simulink model "sm_aileron_actuator_mech_01_ail"  (R2023b)
settings: Solver=VariableStepAuto  StartTime=0.0  StopTime=10.0  RelTol=1e-3  EnableMultiTasking=on
PreLoadFcn:
  | aileronAssembly_DataFile
undefined symbols (not defined in the file): AAC_Param, actbase_x, actbase_y, smiData, X, Y, Z
libraries: sm_lib x303, nesl_utility x1
(part 1 of 6)
Description:
  | Copyright 2018-2022 The MathWorks, Inc.
settings Model: Creator=smiller  LastModifiedBy=mkhaleghi
settings SolverCC: AlgebraicLoopSolver=TrustRegion
settings DataIOCC: LimitDataPoints=on
settings OptimizationCC: ReuseModelBlockBuffer=off  LifeSpan=inf
settings DebuggingCC: UnconnectedInputMsg=warning  UnconnectedOutputMsg=warning  UnconnectedLineMsg=warning  AllowSymbolicDim=off  PregeneratedLibrarySubsystemCodeDiagnostic=none  SFUnexpectedBacktrackingDiag=warning  SFNoUnconditionalDefaultTransitionDiag=warning  SFExecutionAtInitializationDiag=none  ArithmeticOperatorsInVariantConditions=warning
settings ModelReferenceCC: EnableRefExpFcnMdlSchedulingChecks=on
settings SFSimCC: SimUseLocalCustomCode=off  CustomCodeUndefinedFunction=UseInterfaceOnly
settings RTWCC: RTWUseLocalCustomCode=off  DLArmComputeVersion=19.05
settings CodeAppCC: StateflowObjectComments=on
settings GRTTargetCC: TargetLangStandard=C89/C90 (ANSI)
settings ConfigComp: CovMetricSettings=dw  CovSaveCumulativeToWorkspaceVar=on  CovSaveSingleToWorkspaceVar=on  CovExternalEMLEnable=off  CovSFcnEnable=off
settings SimscapeCC: SimscapeNominalValues="[{\"value\":\"10\",\"unit\":\"V\"},{\"value\":\"1\",\"unit\":\"A\"},{\"value\":\"10\",\"unit\":\"N*m\"},{\"value\":\"10\",\"unit\":\"bar\"},{\"value\":\"100\",\"unit\":\"kJ/kg\"},{\"value\":\"1\",\"unit\":\"kW\"},{\"value\":\"300\",\"unit\":\"K\"},{\"value\":\"100\",\"unit\":\"cm^3/s\"},{\"value\":\"1\",\"unit\":\"kN\"},{\"value\":\"1\",\"unit\":\"g/cm^3\"},{\"value\":\"1\",\"unit\":\"l\"},{\"value\":\"1\",\"unit\":\"cm^2\"},{\"value\":\"60\",\"unit\":\"Hz\"}]"  SimscapeLogType=all  SimscapeLogDataHistory=10000
settings ConfigurationSet: Description=SimMechanics 2G
settings ExplorerConfigSet: InternalSimMechanicsExplorerSettings="<ExplorerConfiguration><canonicalview>default</canonicalview><AnimationSetting><BasePlaybackSpeed>1.0</BasePlaybackSpeed><PlaybackSpeedFactor>1.0</PlaybackSpeedFactor></AnimationSetting><TilePanel><TileInfo><Tiles Columns=\"1\" Count=\"1\" Rows=\"1\"><Column Weight=\"1\"/><Row Weight=\"1\"/><Tile Height=\"1\" Width=\"1\" X=\"0\" Y=\"0\"/></Tiles></TileInfo><SceneInfo><SceneViewer><BGColor><R>1</R><G>1</G><B>1</B></BGColor><Camera><DoPerspective>off</DoPerspective><Position><X>0.188789670070064197</X><Y>0.0456123314797882706</Y><Z>3.03630010044172227</Z></Position><Center><X>0.188789670070064197</X><Y>0.0456123314797882706</Y><Z>-0.0389997633735852389</Z></Center><Up><X>0</X><Y>1</Y><Z>-0</Z></Up><ViewLimDist>1</ViewLimDist><YLim>0.256282721906246236</YLim><XLim>0.407121367156505543</XLim></Camera></SceneViewer></SceneInfo></TilePanel><MechEditorPanel><Cameras/><GfxPanelCameraMap/><VideoCreator><PlaybackSpeedRatio>1.0</PlaybackSpeedRatio><FrameRate>30</FrameRate><VideoFormat>Motion JPEG AVI</VideoFormat><FrameSize>auto</FrameSize></VideoCreator></MechEditorPanel></ExplorerConfiguration>"

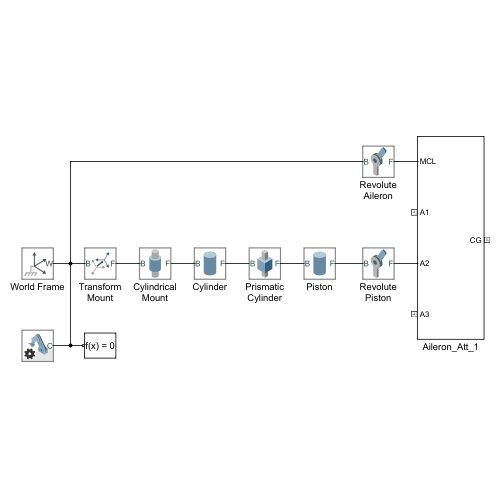
[thumbnail: Simulink's stored preview of the top-level diagram]
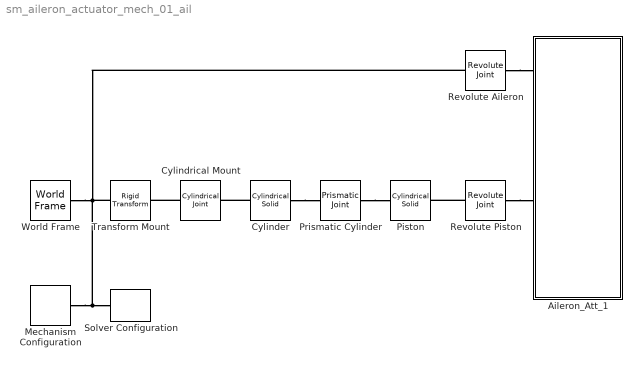
== system sm_aileron_actuator_mech_01_ail ==
  Aileron_Att_1 : Subsystem  RequirementInfo={} %GIDa_f86a7f46_afc1_4b35_ab70_400c1aa97c7d
  Cylinder : sm_lib/Body Elements/Cylindrical Solid  GraphicAmbientColor=[0.15 0.15 0.15 1.0]  BasedOnType=Density  CenterOfMass=[0 0 0]  CenterOfMassUnits=m  GraphicDiffuseColor=[1.0 0.8 0.4]  CylinderLength=cyl_length  CylinderLengthUnits=m  CylinderRadius=cyl_radius  CylinderRadiusUnits=m  Density=1000  DensityUnits=kg/m^3  DoExposeReferenceFrame=off  GraphicEmissiveColor=[0.0 0.0 0.0 1.0]  ExportEntireGeometry=off  SerializedFrames=<Frames><Frame><Id>Frame1</Id><Value><Name>F</Name><Origin><Source>GeometricFeature</Source><FeatureName>top surface</FeatureName></Origin><PrimaryAxis><DefinedDirection>+Z</DefinedDirection><Source>GeometricFeature</Source><SourceDirection>+Z</SourceDirection><FeatureName>top surface</FeatureName></PrimaryAxis><SecondaryAxis><DefinedDirection>+X</DefinedDirection><Source>ReferenceFrame</Source><SourceDirection>+X</SourceDirection><FeatureName></FeatureName></SecondaryAxis></Value></Frame><Frame><Id>Frame2</Id><Value><Name>B</Name><Origin><Source>GeometricFeature</Source><FeatureName>bottom surface</FeatureName></Origin><PrimaryAxis><DefinedDirection>+Z</DefinedDirection><Source>ReferenceFrame</Source><SourceDirection>-X</SourceDirection><FeatureName></FeatureName></PrimaryAxis><SecondaryAxis><DefinedDirection>+X</DefinedDirection><Source>ReferenceFrame</Source><SourceDirection>+Z</SourceDirection><FeatureName></FeatureName></SecondaryAxis></Value></Frame></Frames>  MarkerShape=Sphere  MarkerSize=10  GraphicType=FromGeometry  InertiaType=CalculateFromGeometry  Mass=1  MassUnits=kg  MomentsOfInertia=[1 1 1]  MomentsOfInertiaUnits=kg*m^2  GraphicOpacity=1.0  ProductsOfInertia=[0 0 0]  ProductsOfInertiaUnits=kg*m^2  GraphicShininess=75  GraphicSpecularColor=[0.5 0.5 0.5 1.0]  GraphicVisPropType=SimpleVisualProperties
  Cylindrical Mount : sm_lib/Joints/Cylindrical Joint  JointMode=Normal  SenseConstraintForce=off  SenseConstraintForceX=off  SenseConstraintForceY=off  SenseConstraintForceZ=off  SenseConstraintTorque=off  SenseConstraintTorqueX=off  SenseConstraintTorqueY=off  SenseConstraintTorqueZ=off  SenseTotalForce=off  SenseTotalForceX=off  SenseTotalForceY=off  SenseTotalForceZ=off  SenseTotalTorque=off  SenseTotalTorqueX=off  SenseTotalTorqueY=off  SenseTotalTorqueZ=off  CompositeWrenchDir=FollowerOnBase  CompositeWrenchFrame=BaseFrame  PzEquilibriumPosition=0  PzEquilibriumPositionUnits=m  PzSpringStiffness=0  PzSpringStiffnessUnits=N/m  PzDampingCoefficient=0  PzDampingCoefficientUnits=N/(m/s)  PzTorqueActuationMode=NoTorque  PzMotionActuationMode=ComputedMotion  PzSensePosition=off  PzSenseVelocity=off  PzSenseAcceleration=off  PzSenseTorqueForce=off  PzSenseLowerLimitTorqueForce=off  PzSenseUpperLimitTorqueForce=off  PzLowerLimitSpecify=off  PzLowerLimitBound=-1  PzLowerLimitBoundUnits=m  PzLowerLimitStiffness=1e6  PzLowerLimitStiffnessUnits=N/m  PzLowerLimitDamping=1e3  PzLowerLimitDampingUnits=N/(m/s)  PzLowerLimitTransitionRegionWidth=1e-4  PzLowerLimitTransitionRegionWidthUnits=m  PzUpperLimitSpecify=off  PzUpperLimitBound=1  PzUpperLimitBoundUnits=m  PzUpperLimitStiffness=1e6  PzUpperLimitStiffnessUnits=N/m  PzUpperLimitDamping=1e3  PzUpperLimitDampingUnits=N/(m/s)  PzUpperLimitTransitionRegionWidth=1e-4  PzUpperLimitTransitionRegionWidthUnits=m  PzPositionTargetSpecify=off  PzPositionTargetPriority=High  PzPositionTargetValue=0  PzPositionTargetValueUnits=m  PzVelocityTargetSpecify=off  PzVelocityTargetPriority=High  PzVelocityTargetValue=0  PzVelocityTargetValueUnits=m/s  RzEquilibriumPosition=0  RzEquilibriumPositionUnits=deg  RzSpringStiffness=0  RzSpringStiffnessUnits=N*m/deg  RzDampingCoefficient=0  RzDampingCoefficientUnits=N*m/(deg/s)  RzTorqueActuationMode=NoTorque  RzMotionActuationMode=ComputedMotion  RzSensePosition=off  RzSenseVelocity=off  RzSenseAcceleration=off  RzSenseTorqueForce=off  RzSenseLowerLimitTorqueForce=off  RzSenseUpperLimitTorqueForce=off  RzLowerLimitSpecify=off  RzLowerLimitBound=-90  RzLowerLimitBoundUnits=deg  RzLowerLimitStiffness=1e4  RzLowerLimitStiffnessUnits=N*m/deg  RzLowerLimitDamping=10  RzLowerLimitDampingUnits=N*m/(deg/s)  RzLowerLimitTransitionRegionWidth=0.1  RzLowerLimitTransitionRegionWidthUnits=deg  RzUpperLimitSpecify=off  RzUpperLimitBound=90  RzUpperLimitBoundUnits=deg  RzUpperLimitStiffness=1e4  RzUpperLimitStiffnessUnits=N*m/deg  RzUpperLimitDamping=10  RzUpperLimitDampingUnits=N*m/(deg/s)  RzUpperLimitTransitionRegionWidth=0.1  RzUpperLimitTransitionRegionWidthUnits=deg  RzPositionTargetSpecify=off  RzPositionTargetPriority=High  RzPositionTargetValue=0  RzPositionTargetValueUnits=deg  RzVelocityTargetSpecify=off  RzVelocityTargetPriority=High  RzVelocityTargetValue=0  RzVelocityTargetValueUnits=deg/s
  Mechanism Configuration : sm_lib/Utilities/Mechanism Configuration  UniformGravity=Constant  GravityVector=[0 -9.80665 0]  GravityVectorUnits=m/s^2  LinearizationDelta=0.001  JointModeTransitionNonlinearIterations=2
  Piston : sm_lib/Body Elements/Cylindrical Solid  GraphicAmbientColor=[0.15 0.15 0.15 1.0]  BasedOnType=Density  CenterOfMass=[0 0 0]  CenterOfMassUnits=m  GraphicDiffuseColor=[0.5 0.5 0.5]  CylinderLength=piston_length  CylinderLengthUnits=m  CylinderRadius=piston_radius  CylinderRadiusUnits=m  Density=1000  DensityUnits=kg/m^3  DoExposeReferenceFrame=off  GraphicEmissiveColor=[0.0 0.0 0.0 1.0]  ExportEntireGeometry=off  SerializedFrames=<Frames><Frame><Id>Frame1</Id><Value><Name>F</Name><Origin><Source>GeometricFeature</Source><FeatureName>top surface</FeatureName></Origin><PrimaryAxis><DefinedDirection>+Z</DefinedDirection><Source>ReferenceFrame</Source><SourceDirection>-X</SourceDirection><FeatureName></FeatureName></PrimaryAxis><SecondaryAxis><DefinedDirection>+X</DefinedDirection><Source>ReferenceFrame</Source><SourceDirection>+Z</SourceDirection><FeatureName></FeatureName></SecondaryAxis></Value></Frame><Frame><Id>Frame2</Id><Value><Name>B</Name><Origin><Source>GeometricFeature</Source><FeatureName>bottom surface</FeatureName></Origin><PrimaryAxis><DefinedDirection>+Z</DefinedDirection><Source>ReferenceFrame</Source><SourceDirection>+Z</SourceDirection><FeatureName></FeatureName></PrimaryAxis><SecondaryAxis><DefinedDirection>+X</DefinedDirection><Source>ReferenceFrame</Source><SourceDirection>+X</SourceDirection><FeatureName></FeatureName></SecondaryAxis></Value></Frame></Frames>  MarkerShape=Sphere  MarkerSize=10  GraphicType=FromGeometry  InertiaType=CalculateFromGeometry  Mass=1  MassUnits=kg  MomentsOfInertia=[1 1 1]  MomentsOfInertiaUnits=kg*m^2  GraphicOpacity=1.0  ProductsOfInertia=[0 0 0]  ProductsOfInertiaUnits=kg*m^2  GraphicShininess=75  GraphicSpecularColor=[0.5 0.5 0.5 1.0]  GraphicVisPropType=SimpleVisualProperties
  Prismatic Cylinder : sm_lib/Joints/Prismatic Joint  JointMode=Normal  SenseConstraintForce=off  SenseConstraintForceX=off  SenseConstraintForceY=off  SenseConstraintForceZ=off  SenseConstraintTorque=off  SenseConstraintTorqueX=off  SenseConstraintTorqueY=off  SenseConstraintTorqueZ=off  SenseTotalForce=off  SenseTotalForceX=off  SenseTotalForceY=off  SenseTotalForceZ=off  SenseTotalTorque=off  SenseTotalTorqueX=off  SenseTotalTorqueY=off  SenseTotalTorqueZ=off  CompositeWrenchDir=FollowerOnBase  CompositeWrenchFrame=BaseFrame  EquilibriumPosition=0  EquilibriumPositionUnits=m  SpringStiffness=0  SpringStiffnessUnits=N/m  DampingCoefficient=0  DampingCoefficientUnits=N/(m/s)  TorqueActuationMode=NoTorque  MotionActuationMode=ComputedMotion  SensePosition=off  SenseVelocity=off  SenseAcceleration=off  SenseTorqueForce=off  SenseLowerLimitTorqueForce=off  SenseUpperLimitTorqueForce=off  LowerLimitSpecify=off  LowerLimitBound=-1  LowerLimitBoundUnits=m  LowerLimitStiffness=1e6  LowerLimitStiffnessUnits=N/m  LowerLimitDamping=1e3  LowerLimitDampingUnits=N/(m/s)  LowerLimitTransitionRegionWidth=1e-4  LowerLimitTransitionRegionWidthUnits=m  UpperLimitSpecify=off  UpperLimitBound=1  UpperLimitBoundUnits=m  UpperLimitStiffness=1e6  UpperLimitStiffnessUnits=N/m  UpperLimitDamping=1e3  UpperLimitDampingUnits=N/(m/s)  UpperLimitTransitionRegionWidth=1e-4  UpperLimitTransitionRegionWidthUnits=m  PositionTargetSpecify=off  PositionTargetPriority=High  PositionTargetValue=0  PositionTargetValueUnits=m  VelocityTargetSpecify=off  VelocityTargetPriority=High  VelocityTargetValue=0  VelocityTargetValueUnits=m/s
  Revolute Aileron : sm_lib/Joints/Revolute Joint  JointMode=Normal  SenseConstraintForce=off  SenseConstraintForceX=off  SenseConstraintForceY=off  SenseConstraintForceZ=off  SenseConstraintTorque=off  SenseConstraintTorqueX=off  SenseConstraintTorqueY=off  SenseConstraintTorqueZ=off  SenseTotalForce=off  SenseTotalForceX=off  SenseTotalForceY=off  SenseTotalForceZ=off  SenseTotalTorque=off  SenseTotalTorqueX=off  SenseTotalTorqueY=off  SenseTotalTorqueZ=off  CompositeWrenchDir=FollowerOnBase  CompositeWrenchFrame=BaseFrame  EquilibriumPosition=0  EquilibriumPositionUnits=deg  SpringStiffness=0  SpringStiffnessUnits=N*m/deg  DampingCoefficient=0  DampingCoefficientUnits=N*m/(deg/s)  TorqueActuationMode=NoTorque  MotionActuationMode=ComputedMotion  SensePosition=off  SenseVelocity=off  SenseAcceleration=off  SenseTorqueForce=off  SenseLowerLimitTorqueForce=off  SenseUpperLimitTorqueForce=off  LowerLimitSpecify=off  LowerLimitBound=-90  LowerLimitBoundUnits=deg  LowerLimitStiffness=1e4  LowerLimitStiffnessUnits=N*m/deg  LowerLimitDamping=10  LowerLimitDampingUnits=N*m/(deg/s)  LowerLimitTransitionRegionWidth=0.1  LowerLimitTransitionRegionWidthUnits=deg  UpperLimitSpecify=off  UpperLimitBound=90  UpperLimitBoundUnits=deg  UpperLimitStiffness=1e4  UpperLimitStiffnessUnits=N*m/deg  UpperLimitDamping=10  UpperLimitDampingUnits=N*m/(deg/s)  UpperLimitTransitionRegionWidth=0.1  UpperLimitTransitionRegionWidthUnits=deg  PositionTargetSpecify=on  PositionTargetPriority=High  PositionTargetValue=0  PositionTargetValueUnits=deg  VelocityTargetSpecify=off  VelocityTargetPriority=High  VelocityTargetValue=0  VelocityTargetValueUnits=deg/s
  Revolute Piston : sm_lib/Joints/Revolute Joint  JointMode=Normal  SenseConstraintForce=off  SenseConstraintForceX=off  SenseConstraintForceY=off  SenseConstraintForceZ=off  SenseConstraintTorque=off  SenseConstraintTorqueX=off  SenseConstraintTorqueY=off  SenseConstraintTorqueZ=off  SenseTotalForce=off  SenseTotalForceX=off  SenseTotalForceY=off  SenseTotalForceZ=off  SenseTotalTorque=off  SenseTotalTorqueX=off  SenseTotalTorqueY=off  SenseTotalTorqueZ=off  CompositeWrenchDir=FollowerOnBase  CompositeWrenchFrame=BaseFrame  EquilibriumPosition=0  EquilibriumPositionUnits=deg  SpringStiffness=0  SpringStiffnessUnits=N*m/deg  DampingCoefficient=0  DampingCoefficientUnits=N*m/(deg/s)  TorqueActuationMode=NoTorque  MotionActuationMode=ComputedMotion  SensePosition=off  SenseVelocity=off  SenseAcceleration=off  SenseTorqueForce=off  SenseLowerLimitTorqueForce=off  SenseUpperLimitTorqueForce=off  LowerLimitSpecify=off  LowerLimitBound=-90  LowerLimitBoundUnits=deg  LowerLimitStiffness=1e4  LowerLimitStiffnessUnits=N*m/deg  LowerLimitDamping=10  LowerLimitDampingUnits=N*m/(deg/s)  LowerLimitTransitionRegionWidth=0.1  LowerLimitTransitionRegionWidthUnits=deg  UpperLimitSpecify=off  UpperLimitBound=90  UpperLimitBoundUnits=deg  UpperLimitStiffness=1e4  UpperLimitStiffnessUnits=N*m/deg  UpperLimitDamping=10  UpperLimitDampingUnits=N*m/(deg/s)  UpperLimitTransitionRegionWidth=0.1  UpperLimitTransitionRegionWidthUnits=deg  PositionTargetSpecify=off  PositionTargetPriority=High  PositionTargetValue=0  PositionTargetValueUnits=deg  VelocityTargetSpecify=off  VelocityTargetPriority=High  VelocityTargetValue=0  VelocityTargetValueUnits=deg/s
  Solver Configuration : nesl_utility/Solver Configuration  PhysicalDomain=network_engine_domain  SubClassName=solver  LeftPortType=input  RightPortType=generic  Tones=[]  Harmonics=[]  SimulateNoise=off  Profile=off  UseLocalSampling=off  EnableSwitchedLinearOptims=on  FrequencyDomain=off  UseCCode=off  RelTol=0.001  AbsTol=1e-06  MinStep=1e-09  ToWorkspace=off  RevertToSquareIcSolve=off  NumHomotopyIterations=100  PhasorMode=off  PhasorModeNumHarmonics=1  ConsistencySolver=NEWTON_XTOL_AFTER_FTOL  IndexReductionMethod=DerivativeReplacement  DoDC=off  ResidualTolerance=1e-09  ConsistencyTolSource=GLOBAL  ConsistencyAbsTol=0.001  ConsistencyRelTol=0.001  ConsistencyTolFactor=0.001  UseLocalSolver=off  LocalSolverChoice=NE_BACKWARD_EULER_ADVANCER  ResolveIndetEquations=on  FunctionEvalNumThread=1  LocalSolverSampleTime=0.001  DoFixedCost=off  MaxNonlinIter=3  MaxModeIter=2  ComputeImpulses=off  ImpulseIterations=2  LinearAlgebra=Sparse  LinearAlgebraNumThread=0  EquationFormulation=NE_TIME_EF  DelaysMemoryBudget=1024  AutomaticFiltering=on  FilteringTimeConstant=0.001  PartitionStorageMethod=AS_NEEDED  PartitionMemoryBudget=1024  PartitionMethod=FAST  MultibodyUseLocalSolver=off  MultibodyLocalSolverChoice=ODE1  MultibodyLocalSolverSampleTime=0.001
  Transform Mount : sm_lib/Frames and Transforms/Rigid Transform  TranslationMethod=Cartesian  TranslationStandardOffset=0.4  TranslationStandardOffsetUnits=m  TranslationStandardAxis=-X  TranslationCartesianOffset=[actbase_x actbase_y 0]  TranslationCartesianOffsetUnits=m  TranslationROffset=0  TranslationROffsetUnits=m  TranslationZOffset=0  TranslationZOffsetUnits=m  TranslationThetaOffset=0  TranslationThetaOffsetUnits=deg  RotationMethod=None  RotationAngleUnits=deg  RotationStandardAxis=+Z  RotationAngle=0.0  RotationArbitraryAxis=[0 0 1]  FollAlignAxisA=+X  BaseAlignAxisA=+Y  FollAlignAxisB=+Y  BaseAlignAxisB=+Z  RotationSequenceAxes=FollowerAxes  RotationSequence=XYX  RotationSequenceAngles=[0 0 0]  RotationSequenceAnglesUnits=deg  RotationMatrix=[1 0 0; 0 1 0; 0 0 1]  Quaternion=[1 0 0 0]
  World Frame : sm_lib/Frames and Transforms/World Frame
  connections:
  Mechanism Configuration/RConn1 -- Revolute Aileron/LConn1 -- World Frame/RConn1 -- Transform Mount/LConn1 -- Solver Configuration/RConn1
  Revolute Aileron/RConn1 -- Aileron_Att_1/LConn1
  Revolute Piston/RConn1 -- Aileron_Att_1/LConn3
  Revolute Piston/LConn1 -- Piston/LConn1
  Prismatic Cylinder/RConn1 -- Piston/RConn1
  Cylinder/LConn1 -- Prismatic Cylinder/LConn1
  Cylindrical Mount/LConn1 -- Transform Mount/RConn1
  Cylinder/RConn1 -- Cylindrical Mount/RConn1

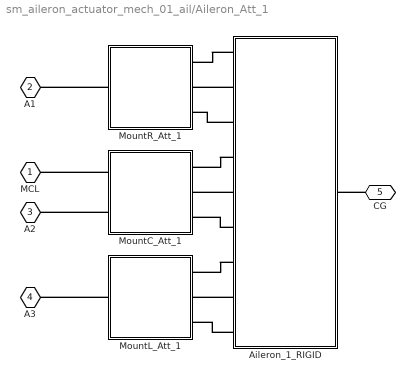
== system sm_aileron_actuator_mech_01_ail/Aileron_Att_1 ==
  Aileron_1_RIGID : Subsystem  RequirementInfo={} %GIDa_49195487_d7f9_40de_a207_408c1accc14d
  MountC_Att_1 : Subsystem  RequirementInfo={} %GIDa_cc448e52_c2f2_42ee_93a5_1fa9538c0a17
  MountL_Att_1 : Subsystem  RequirementInfo={} %GIDa_6a0c2f59_c236_42a3_9b97_8a4534d6f5fc
  MountR_Att_1 : Subsystem  RequirementInfo={} %GIDa_ba62e863_ceca_4ebe_b6f4_5b9dac20edd9
  MCL : PMIOPort  RequirementInfo={} %GIDa_50b812aa_efc3_46e4_8f02_72f1b4dd47f6  Side=Left
  A1 : PMIOPort  RequirementInfo={} %GIDa_90595992_d13c_4b76_abe8_99ed1bc53ea1  Port=2  Side=Left
  A2 : PMIOPort  RequirementInfo={} %GIDa_199c94c7_d645_4e17_a3c1_0716841b5a25  Port=3  Side=Left
  A3 : PMIOPort  RequirementInfo={} %GIDa_7d780e1c_4259_4ce4_9e0e_7a2c492cfa8f  Port=4  Side=Left
  CG : PMIOPort  RequirementInfo={} %GIDa_58d05848_c354_4c6c_a441_548dc6264d86  Port=5  Side=Right
  connections:
  Aileron_1_RIGID/LConn5 -- MountC_Att_1/RConn2
  Aileron_1_RIGID/LConn6 -- MountC_Att_1/RConn3
  MountC_Att_1/LConn1 -- MCL/RConn1
  MountC_Att_1/LConn2 -- A2/RConn1
  MountL_Att_1/LConn1 -- A3/RConn1
  Aileron_1_RIGID/LConn4 -- MountC_Att_1/RConn1
  Aileron_1_RIGID/LConn1 -- MountR_Att_1/RConn1
  Aileron_1_RIGID/LConn3 -- MountR_Att_1/RConn3
  Aileron_1_RIGID/LConn2 -- MountR_Att_1/RConn2
  Aileron_1_RIGID/LConn9 -- MountL_Att_1/RConn3
  Aileron_1_RIGID/LConn8 -- MountL_Att_1/RConn2
  Aileron_1_RIGID/LConn7 -- MountL_Att_1/RConn1
  MountR_Att_1/LConn1 -- A1/RConn1
  CG/RConn1 -- Aileron_1_RIGID/RConn1

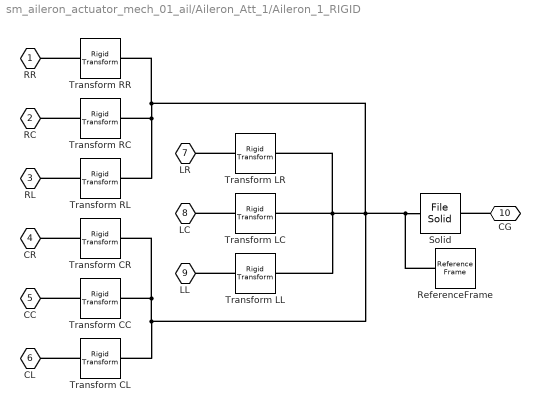
== system sm_aileron_actuator_mech_01_ail/Aileron_Att_1/Aileron_1_RIGID ==
  ReferenceFrame : sm_lib/Frames and Transforms/Reference Frame  RequirementInfo={} %GIDa_21f32e3a_5f71_4ee6_96e7_2de100356797
  Solid : sm_lib/Body Elements/File Solid  RequirementInfo={} %GIDa_922de579_a86a_4404_a1e8_cb4817ddeba3  ExtGeomFileName=Aileron.step  UnitType=FromFile  ExtGeomFileUnits=m  StepReaderType=HEX  ExportConvexHullGeometry=off  InertiaType=Custom  Mass=smiData.Solid(9).mass  MassUnits=kg  CenterOfMass=smiData.Solid(9).CoM  CenterOfMassUnits=m  MomentsOfInertia=smiData.Solid(9).MoI  MomentsOfInertiaUnits=kg*m^2  ProductsOfInertia=smiData.Solid(9).PoI  ProductsOfInertiaUnits=kg*m^2  BasedOnType=Density  Density=1000  DensityUnits=kg/m^3  DoExposeReferenceFrame=on  SerializedFrames=<Frames><Frame><Id>Frame1</Id><Value><Name>CG</Name><Origin><Source>CenterOfMassFrame</Source><FeatureName></FeatureName></Origin><PrimaryAxis><DefinedDirection>+Z</DefinedDirection><Source>ReferenceFrame</Source><SourceDirection>+Z</SourceDirection><FeatureName></FeatureName></PrimaryAxis><SecondaryAxis><DefinedDirection>+X</DefinedDirection><Source>ReferenceFrame</Source><SourceDirection>+X</SourceDirection><FeatureName></FeatureName></SecondaryAxis></Value></Frame></Frames>  GraphicType=FromGeometry  MarkerShape=Sphere  MarkerSize=10  GraphicVisPropType=SimpleVisualProperties  GraphicDiffuseColor=smiData.Solid(9).color  GraphicSpecularColor=[0.5 0.5 0.5 1.0]  GraphicAmbientColor=[0.15 0.15 0.15 1.0]  GraphicEmissiveColor=[0.0 0.0 0.0 1.0]  GraphicShininess=75  GraphicOpacity=smiData.Solid(9).opacity*0.5
  Transform CC : sm_lib/Frames and Transforms/Rigid Transform  RequirementInfo={} %GIDa_ebd8302c_e458_43ba_8371_06265ccdad24  TranslationMethod=Cartesian  TranslationStandardOffset=0  TranslationStandardOffsetUnits=m  TranslationStandardAxis=+Z  TranslationCartesianOffset=smiData.RigidTransform(171).translation  TranslationCartesianOffsetUnits=m  TranslationROffset=0  TranslationROffsetUnits=m  TranslationZOffset=0  TranslationZOffsetUnits=m  TranslationThetaOffset=0  TranslationThetaOffsetUnits=deg  RotationMethod=ArbitraryAxis  RotationAngleUnits=rad  RotationStandardAxis=+Z  RotationAngle=smiData.RigidTransform(171).angle  RotationArbitraryAxis=smiData.RigidTransform(171).axis  FollAlignAxisA=+X  BaseAlignAxisA=+Y  FollAlignAxisB=+Y  BaseAlignAxisB=+Z  RotationSequenceAxes=FollowerAxes  RotationSequence=XYX  RotationSequenceAngles=[0 0 0]  RotationSequenceAnglesUnits=deg  RotationMatrix=[1 0 0; 0 1 0; 0 0 1]  Quaternion=[1 0 0 0]
  Transform CL : sm_lib/Frames and Transforms/Rigid Transform  RequirementInfo={} %GIDa_acc2fa92_2bec_4f5f_bb9e_37ccad3455bd  TranslationMethod=Cartesian  TranslationStandardOffset=0  TranslationStandardOffsetUnits=m  TranslationStandardAxis=+Z  TranslationCartesianOffset=smiData.RigidTransform(173).translation  TranslationCartesianOffsetUnits=m  TranslationROffset=0  TranslationROffsetUnits=m  TranslationZOffset=0  TranslationZOffsetUnits=m  TranslationThetaOffset=0  TranslationThetaOffsetUnits=deg  RotationMethod=ArbitraryAxis  RotationAngleUnits=rad  RotationStandardAxis=+Z  RotationAngle=smiData.RigidTransform(173).angle  RotationArbitraryAxis=smiData.RigidTransform(173).axis  FollAlignAxisA=+X  BaseAlignAxisA=+Y  FollAlignAxisB=+Y  BaseAlignAxisB=+Z  RotationSequenceAxes=FollowerAxes  RotationSequence=XYX  RotationSequenceAngles=[0 0 0]  RotationSequenceAnglesUnits=deg  RotationMatrix=[1 0 0; 0 1 0; 0 0 1]  Quaternion=[1 0 0 0]
  Transform CR : sm_lib/Frames and Transforms/Rigid Transform  RequirementInfo={} %GIDa_c9b7ffd0_919c_4c82_98d9_b367c221b2bc  TranslationMethod=Cartesian  TranslationStandardOffset=0  TranslationStandardOffsetUnits=m  TranslationStandardAxis=+Z  TranslationCartesianOffset=smiData.RigidTransform(175).translation  TranslationCartesianOffsetUnits=m  TranslationROffset=0  TranslationROffsetUnits=m  TranslationZOffset=0  TranslationZOffsetUnits=m  TranslationThetaOffset=0  TranslationThetaOffsetUnits=deg  RotationMethod=ArbitraryAxis  RotationAngleUnits=rad  RotationStandardAxis=+Z  RotationAngle=smiData.RigidTransform(175).angle  RotationArbitraryAxis=smiData.RigidTransform(175).axis  FollAlignAxisA=+X  BaseAlignAxisA=+Y  FollAlignAxisB=+Y  BaseAlignAxisB=+Z  RotationSequenceAxes=FollowerAxes  RotationSequence=XYX  RotationSequenceAngles=[0 0 0]  RotationSequenceAnglesUnits=deg  RotationMatrix=[1 0 0; 0 1 0; 0 0 1]  Quaternion=[1 0 0 0]
  Transform LC : sm_lib/Frames and Transforms/Rigid Transform  RequirementInfo={} %GIDa_56eade6f_3072_45c6_9e93_f296c845332f  TranslationMethod=Cartesian  TranslationStandardOffset=0  TranslationStandardOffsetUnits=m  TranslationStandardAxis=+Z  TranslationCartesianOffset=smiData.RigidTransform(186).translation  TranslationCartesianOffsetUnits=m  TranslationROffset=0  TranslationROffsetUnits=m  TranslationZOffset=0  TranslationZOffsetUnits=m  TranslationThetaOffset=0  TranslationThetaOffsetUnits=deg  RotationMethod=ArbitraryAxis  RotationAngleUnits=rad  RotationStandardAxis=+Z  RotationAngle=smiData.RigidTransform(186).angle  RotationArbitraryAxis=smiData.RigidTransform(186).axis  FollAlignAxisA=+X  BaseAlignAxisA=+Y  FollAlignAxisB=+Y  BaseAlignAxisB=+Z  RotationSequenceAxes=FollowerAxes  RotationSequence=XYX  RotationSequenceAngles=[0 0 0]  RotationSequenceAnglesUnits=deg  RotationMatrix=[1 0 0; 0 1 0; 0 0 1]  Quaternion=[1 0 0 0]
  Transform LL : sm_lib/Frames and Transforms/Rigid Transform  RequirementInfo={} %GIDa_98338c26_0631_4e74_9043_f68f203014db  TranslationMethod=Cartesian  TranslationStandardOffset=0  TranslationStandardOffsetUnits=m  TranslationStandardAxis=+Z  TranslationCartesianOffset=smiData.RigidTransform(184).translation  TranslationCartesianOffsetUnits=m  TranslationROffset=0  TranslationROffsetUnits=m  TranslationZOffset=0  TranslationZOffsetUnits=m  TranslationThetaOffset=0  TranslationThetaOffsetUnits=deg  RotationMethod=ArbitraryAxis  RotationAngleUnits=rad  RotationStandardAxis=+Z  RotationAngle=smiData.RigidTransform(184).angle  RotationArbitraryAxis=smiData.RigidTransform(184).axis  FollAlignAxisA=+X  BaseAlignAxisA=+Y  FollAlignAxisB=+Y  BaseAlignAxisB=+Z  RotationSequenceAxes=FollowerAxes  RotationSequence=XYX  RotationSequenceAngles=[0 0 0]  RotationSequenceAnglesUnits=deg  RotationMatrix=[1 0 0; 0 1 0; 0 0 1]  Quaternion=[1 0 0 0]
  Transform LR : sm_lib/Frames and Transforms/Rigid Transform  RequirementInfo={} %GIDa_5a6fb82e_5763_4f1b_8260_566eab0c080a  TranslationMethod=Cartesian  TranslationStandardOffset=0  TranslationStandardOffsetUnits=m  TranslationStandardAxis=+Z  TranslationCartesianOffset=smiData.RigidTransform(188).translation  TranslationCartesianOffsetUnits=m  TranslationROffset=0  TranslationROffsetUnits=m  TranslationZOffset=0  TranslationZOffsetUnits=m  TranslationThetaOffset=0  TranslationThetaOffsetUnits=deg  RotationMethod=ArbitraryAxis  RotationAngleUnits=rad  RotationStandardAxis=+Z  RotationAngle=smiData.RigidTransform(188).angle  RotationArbitraryAxis=smiData.RigidTransform(188).axis  FollAlignAxisA=+X  BaseAlignAxisA=+Y  FollAlignAxisB=+Y  BaseAlignAxisB=+Z  RotationSequenceAxes=FollowerAxes  RotationSequence=XYX  RotationSequenceAngles=[0 0 0]  RotationSequenceAnglesUnits=deg  RotationMatrix=[1 0 0; 0 1 0; 0 0 1]  Quaternion=[1 0 0 0]
  Transform RC : sm_lib/Frames and Transforms/Rigid Transform  RequirementInfo={} %GIDa_d1a4983b_b47d_4a82_b8af_8e24d4d9712b  TranslationMethod=Cartesian  TranslationStandardOffset=0  TranslationStandardOffsetUnits=m  TranslationStandardAxis=+Z  TranslationCartesianOffset=smiData.RigidTransform(182).translation  TranslationCartesianOffsetUnits=m  TranslationROffset=0  TranslationROffsetUnits=m  TranslationZOffset=0  TranslationZOffsetUnits=m  TranslationThetaOffset=0  TranslationThetaOffsetUnits=deg  RotationMethod=ArbitraryAxis  RotationAngleUnits=rad  RotationStandardAxis=+Z  RotationAngle=smiData.RigidTransform(182).angle  RotationArbitraryAxis=smiData.RigidTransform(182).axis  FollAlignAxisA=+X  BaseAlignAxisA=+Y  FollAlignAxisB=+Y  BaseAlignAxisB=+Z  RotationSequenceAxes=FollowerAxes  RotationSequence=XYX  RotationSequenceAngles=[0 0 0]  RotationSequenceAnglesUnits=deg  RotationMatrix=[1 0 0; 0 1 0; 0 0 1]  Quaternion=[1 0 0 0]
  Transform RL : sm_lib/Frames and Transforms/Rigid Transform  RequirementInfo={} %GIDa_ab601f74_1be8_4a0a_9190_5f188abf7c1c  TranslationMethod=Cartesian  TranslationStandardOffset=0  TranslationStandardOffsetUnits=m  TranslationStandardAxis=+Z  TranslationCartesianOffset=smiData.RigidTransform(180).translation  TranslationCartesianOffsetUnits=m  TranslationROffset=0  TranslationROffsetUnits=m  TranslationZOffset=0  TranslationZOffsetUnits=m  TranslationThetaOffset=0  TranslationThetaOffsetUnits=deg  RotationMethod=ArbitraryAxis  RotationAngleUnits=rad  RotationStandardAxis=+Z  RotationAngle=smiData.RigidTransform(180).angle  RotationArbitraryAxis=smiData.RigidTransform(180).axis  FollAlignAxisA=+X  BaseAlignAxisA=+Y  FollAlignAxisB=+Y  BaseAlignAxisB=+Z  RotationSequenceAxes=FollowerAxes  RotationSequence=XYX  RotationSequenceAngles=[0 0 0]  RotationSequenceAnglesUnits=deg  RotationMatrix=[1 0 0; 0 1 0; 0 0 1]  Quaternion=[1 0 0 0]
  Transform RR : sm_lib/Frames and Transforms/Rigid Transform  RequirementInfo={} %GIDa_a663f9c1_3ae1_41d3_b3a1_fa442f165817  TranslationMethod=Cartesian  TranslationStandardOffset=0  TranslationStandardOffsetUnits=m  TranslationStandardAxis=+Z  TranslationCartesianOffset=smiData.RigidTransform(177).translation  TranslationCartesianOffsetUnits=m  TranslationROffset=0  TranslationROffsetUnits=m  TranslationZOffset=0  TranslationZOffsetUnits=m  TranslationThetaOffset=0  TranslationThetaOffsetUnits=deg  RotationMethod=ArbitraryAxis  RotationAngleUnits=rad  RotationStandardAxis=+Z  RotationAngle=smiData.RigidTransform(177).angle  RotationArbitraryAxis=smiData.RigidTransform(177).axis  FollAlignAxisA=+X  BaseAlignAxisA=+Y  FollAlignAxisB=+Y  BaseAlignAxisB=+Z  RotationSequenceAxes=FollowerAxes  RotationSequence=XYX  RotationSequenceAngles=[0 0 0]  RotationSequenceAnglesUnits=deg  RotationMatrix=[1 0 0; 0 1 0; 0 0 1]  Quaternion=[1 0 0 0]
  RR : PMIOPort  RequirementInfo={} %GIDa_6d646821_344b_42ea_966c_88088d3bd660  Side=Left
  RC : PMIOPort  RequirementInfo={} %GIDa_73c0888c_d08a_4ab8_a203_4436e9a3b389  Port=2  Side=Left
  RL : PMIOPort  RequirementInfo={} %GIDa_45a8da75_869a_491e_aa98_efb8604524d3  Port=3  Side=Left
  CR : PMIOPort  RequirementInfo={} %GIDa_c438ccf7_87aa_44fc_b1f8_9ab35e406893  Port=4  Side=Left
  CC : PMIOPort  RequirementInfo={} %GIDa_47ef20ac_755f_4f61_be3d_369a8dbfc820  Port=5  Side=Left
  CL : PMIOPort  RequirementInfo={} %GIDa_4cdb6ea3_ef73_4dab_a356_4f4f4f7f5b6b  Port=6  Side=Left
  LR : PMIOPort  RequirementInfo={} %GIDa_ae47e635_f27f_4d80_bb46_5e7b41387957  Port=7  Side=Left
  LC : PMIOPort  RequirementInfo={} %GIDa_a576af36_2119_4284_be19_56222870ba18  Port=8  Side=Left
  LL : PMIOPort  RequirementInfo={} %GIDa_bdfcc04f_d28a_412a_9770_a35fa89f19e7  Port=9  Side=Left
  CG : PMIOPort  RequirementInfo={} %GIDa_4ddf6937_109a_45df_8f9a_5e0855ee7d4a  Port=10  Side=Right
  connections:
  ReferenceFrame/RConn1 -- Transform CR/LConn1 -- Transform CC/LConn1 -- Transform CL/LConn1 -- Transform LL/LConn1 -- Transform LC/LConn1 -- Transform LR/LConn1 -- Transform RL/LConn1 -- Transform RC/LConn1 -- Transform RR/LConn1 -- Solid/RConn1
  Transform CC/RConn1 -- CC/RConn1
  Transform CL/RConn1 -- CL/RConn1
  Transform CR/RConn1 -- CR/RConn1
  Transform RR/RConn1 -- RR/RConn1
  Transform RL/RConn1 -- RL/RConn1
  Transform RC/RConn1 -- RC/RConn1
  Transform LL/RConn1 -- LL/RConn1
  Transform LC/RConn1 -- LC/RConn1
  Transform LR/RConn1 -- LR/RConn1
  CG/RConn1 -- Solid/LConn1

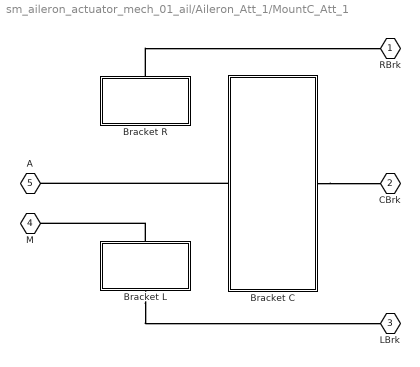
== system sm_aileron_actuator_mech_01_ail/Aileron_Att_1/MountC_Att_1 ==
  Bracket C : Subsystem  RequirementInfo={} %GIDa_df048b02_5fc7_49db_95b2_77d25c86503c
  Bracket L : Subsystem  RequirementInfo={} %GIDa_f33362ec_0cc5_4f07_94e3_9d265febfaed
  Bracket R : Subsystem  RequirementInfo={} %GIDa_b9eb9269_5442_4c0c_9212_2cde85bcb406
  RBrk : PMIOPort  RequirementInfo={} %GIDa_210e43f5_623a_470f_96ee_89fe70a810d3  Side=Right
  CBrk : PMIOPort  RequirementInfo={} %GIDa_28cf98db_3459_4493_8df2_6fa10b41bdf4  Port=2  Side=Right
  LBrk : PMIOPort  RequirementInfo={} %GIDa_c799f118_7fe1_4614_8c34_8e87188f04a7  Port=3  Side=Right
  M : PMIOPort  RequirementInfo={} %GIDa_385b69e7_1f34_408c_a3a8_d2450e4dcc66  Port=4  Side=Left
  A : PMIOPort  RequirementInfo={} %GIDa_35cece3a_3a62_429a_934c_0938af57713d  Port=5  Side=Left
  connections:
  Bracket L/LConn1 -- M/RConn1
  Bracket L/RConn1 -- LBrk/RConn1
  Bracket C/RConn1 -- CBrk/RConn1
  Bracket C/LConn1 -- A/RConn1
  Bracket R/RConn1 -- RBrk/RConn1

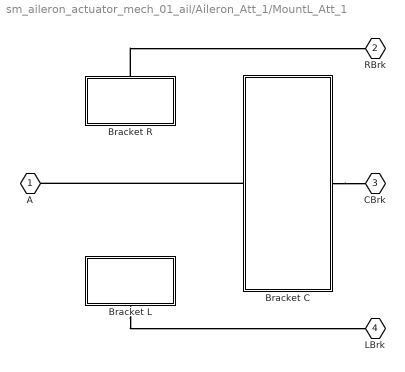
== system sm_aileron_actuator_mech_01_ail/Aileron_Att_1/MountL_Att_1 ==
  Bracket C : Subsystem  RequirementInfo={} %GIDa_4dd0fd38_da53_45b5_b332_2b8b74ef75de
  Bracket L : Subsystem  RequirementInfo={} %GIDa_89d4cec4_2e46_447f_8b59_be2ffb55c735
  Bracket R : Subsystem  RequirementInfo={} %GIDa_9f6b2241_17fe_4487_bf67_dab764f43063
  A : PMIOPort  RequirementInfo={} %GIDa_71a12489_9e6c_4945_8ca6_cee553d0ce2a  Side=Left
  RBrk : PMIOPort  RequirementInfo={} %GIDa_b92cd235_e9e7_4c3d_8e9c_0c736584c72e  Port=2  Side=Right
  CBrk : PMIOPort  RequirementInfo={} %GIDa_5279149f_b496_4bfa_ac7a_6ffe8018919a  Port=3  Side=Right
  LBrk : PMIOPort  RequirementInfo={} %GIDa_a9bfb48b_fbcb_4529_b4a8_933a479a5fcb  Port=4  Side=Right
  connections:
  Bracket C/RConn1 -- CBrk/RConn1
  Bracket C/LConn1 -- A/RConn1
  Bracket L/RConn1 -- LBrk/RConn1
  Bracket R/RConn1 -- RBrk/RConn1

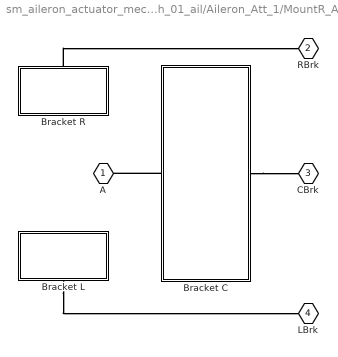
== system sm_aileron_actuator_mech_01_ail/Aileron_Att_1/MountR_Att_1 ==
  Bracket C : Subsystem  RequirementInfo={} %GIDa_c804dd6f_d550_40ae_9040_2f8fa5dec12a
  Bracket L : Subsystem  RequirementInfo={} %GIDa_fa6ca378_34ba_427d_bb91_5f6fbf02c084
  Bracket R : Subsystem  RequirementInfo={} %GIDa_b00dc483_a661_4938_a883_32eade1348ae
  A : PMIOPort  RequirementInfo={} %GIDa_51fe992f_b30d_4c07_870a_e5d95cc069ec  Side=Left
  RBrk : PMIOPort  RequirementInfo={} %GIDa_aa5e2f0b_7e3c_4b43_85c4_7b9b7463d72e  Port=2  Side=Right
  CBrk : PMIOPort  RequirementInfo={} %GIDa_b74934aa_70b7_431a_9eac_8d480ceb934d  Port=3  Side=Right
  LBrk : PMIOPort  RequirementInfo={} %GIDa_ad5b9174_f03b_45df_854f_0a345c0589ea  Port=4  Side=Right
  connections:
  Bracket C/RConn1 -- CBrk/RConn1
  Bracket C/LConn1 -- A/RConn1
  Bracket L/RConn1 -- LBrk/RConn1
  Bracket R/RConn1 -- RBrk/RConn1

== system sm_aileron_actuator_mech_01_ail/Aileron_Att_1/MountC_Att_1/Bracket C ==
  AilBrk_C_1_RIGID : Subsystem  RequirementInfo={} %GIDa_a5eb05cb_6677_40ce_a787_020c8cd855da
  Bolt CBrk : Subsystem  RequirementInfo={} %GIDa_f08550af_5a4a_4263_ba43_4dc158b6f0ea
  Screws CBrk : Subsystem  RequirementInfo={} %GIDa_32458df4_556d_437f_ae65_367062e50304
  Ail : PMIOPort  RequirementInfo={} %GIDa_567b7a60_56b8_4f7a_8d91_20db37820f26  Side=Right
  Act : PMIOPort  RequirementInfo={} %GIDa_a27a7454_fa6a_42d3_a6b5_bfcd69a5d859  Port=2  Side=Left
  connections:
  AilBrk_C_1_RIGID/LConn1 -- Screws CBrk/LConn1 -- Bolt CBrk/LConn1
  AilBrk_C_1_RIGID/RConn1 -- Ail/RConn1
  AilBrk_C_1_RIGID/LConn2 -- Act/RConn1

== system sm_aileron_actuator_mech_01_ail/Aileron_Att_1/MountC_Att_1/Bracket L ==
  AilBrk_L_1_RIGID : Subsystem  RequirementInfo={} %GIDa_651b5bea_d620_4abf_82a1_83d0a1186e81
  Bolt LBrk : Subsystem  RequirementInfo={} %GIDa_3b4d410c_9a3d_4d47_8ce3_69012dd8230c
  Screws LBrk : Subsystem  RequirementInfo={} %GIDa_4ad5ce10_7b21_45e7_890d_ad5afdb9c41e
  M : PMIOPort  RequirementInfo={} %GIDa_b4be3496_a9c2_4fa2_8781_c9d27c8b9ad6  Side=Left
  Ail : PMIOPort  RequirementInfo={} %GIDa_606ac865_fcca_4608_a4a3_3911e104ff5a  Port=2  Side=Right
  connections:
  Screws LBrk/LConn1 -- Bolt LBrk/LConn2 -- AilBrk_L_1_RIGID/LConn1
  Bolt LBrk/LConn1 -- M/RConn1
  AilBrk_L_1_RIGID/RConn1 -- Ail/RConn1

== system sm_aileron_actuator_mech_01_ail/Aileron_Att_1/MountC_Att_1/Bracket R ==
  AilBrk_R_1_RIGID : Subsystem  RequirementInfo={} %GIDa_424add49_065e_41fb_992e_ec5f6f59f4a7
  Bolt RBrk : Subsystem  RequirementInfo={} %GIDa_02499ea9_2854_43d2_9a9c_a6c4b9010727
  Screws RBrk : Subsystem  RequirementInfo={} %GIDa_625b1a6d_8f2d_46c5_8154_3bb31bfd7cd0
  Ail : PMIOPort  RequirementInfo={} %GIDa_2cae7c5f_ffb7_4077_8ca2_3662fb4fa6ed  Side=Right
  connections:
  AilBrk_R_1_RIGID/LConn1 -- Screws RBrk/LConn1 -- Bolt RBrk/LConn1
  AilBrk_R_1_RIGID/RConn1 -- Ail/RConn1

== system sm_aileron_actuator_mech_01_ail/Aileron_Att_1/MountL_Att_1/Bracket C ==
  AilBrk_C_1_RIGID : Subsystem  RequirementInfo={} %GIDa_dbf9ed39_f1e5_4564_a20b_5265f8e90a94
  Bolt CBrk : Subsystem  RequirementInfo={} %GIDa_3b4dd506_366a_48b6_81a9_b6e5c6efc659
  Screws CBrk : Subsystem  RequirementInfo={} %GIDa_944ca8ff_809d_4111_b3a8_2083901704c5
  Ail : PMIOPort  RequirementInfo={} %GIDa_713fc6a2_5b59_4a98_a307_c1d4e987e334  Side=Right
  Act : PMIOPort  RequirementInfo={} %GIDa_3becd23b_86f9_4fbc_b95a_441888116672  Port=2  Side=Left
  connections:
  AilBrk_C_1_RIGID/LConn1 -- Screws CBrk/LConn1 -- Bolt CBrk/LConn1
  AilBrk_C_1_RIGID/LConn2 -- Act/RConn1
  AilBrk_C_1_RIGID/RConn1 -- Ail/RConn1

== system sm_aileron_actuator_mech_01_ail/Aileron_Att_1/MountL_Att_1/Bracket L ==
  AilBrk_L_1_RIGID : Subsystem  RequirementInfo={} %GIDa_36d9c6bf_1fd9_48c2_97fa_17444e5b7c07
  Bolt LBrk : Subsystem  RequirementInfo={} %GIDa_96f5dace_a0d6_4f26_a0e3_434b09d7727a
  "Screws LBrk " : Subsystem  RequirementInfo={} %GIDa_31c74e47_8913_422a_a8eb_3ab247e389eb
  Ail : PMIOPort  RequirementInfo={} %GIDa_5dfad836_3c14_405d_82ce_b32c75c8a335  Side=Right
  connections:
  AilBrk_L_1_RIGID/LConn1 -- "Screws LBrk "/LConn1 -- Bolt LBrk/LConn1
  AilBrk_L_1_RIGID/RConn1 -- Ail/RConn1

== system sm_aileron_actuator_mech_01_ail/Aileron_Att_1/MountL_Att_1/Bracket R ==
  AilBrk_R_1_RIGID : Subsystem  RequirementInfo={} %GIDa_7c37eec9_8ac7_4455_ad51_87a703a312a9
  Bolt RBrk : Subsystem  RequirementInfo={} %GIDa_bfeebd55_8b98_4e87_92ae_f7606a22fab8
  Screws RBrk : Subsystem  RequirementInfo={} %GIDa_ee5acb61_291c_418d_b62e_9f995e7f0029
  Ail : PMIOPort  RequirementInfo={} %GIDa_0d11db7e_7170_4aa1_9472_3275fb90983b  Side=Right
  connections:
  AilBrk_R_1_RIGID/LConn1 -- Screws RBrk/LConn1 -- Bolt RBrk/LConn1
  AilBrk_R_1_RIGID/RConn1 -- Ail/RConn1

== system sm_aileron_actuator_mech_01_ail/Aileron_Att_1/MountR_Att_1/Bracket C ==
  AilBrk_C_1_RIGID : Subsystem  RequirementInfo={} %GIDa_ec32f1fb_af89_4dba_9142_3966752762f3
  Bolt CBrk : Subsystem  RequirementInfo={} %GIDa_13e331c4_a24d_49d0_b4af_22e8e69b712e
  Screws CBrk : Subsystem  RequirementInfo={} %GIDa_78db7ebf_366c_45a0_a6d8_0d6769ee52cf
  Ail : PMIOPort  RequirementInfo={} %GIDa_fbedc1f1_8c3f_43e9_a54e_4d43f0a4fc34  Side=Right
  Act : PMIOPort  RequirementInfo={} %GIDa_386ca5d9_9175_4713_863c_2ea824254130  Port=2  Side=Left
  connections:
  AilBrk_C_1_RIGID/LConn1 -- Screws CBrk/LConn1 -- Bolt CBrk/LConn1
  AilBrk_C_1_RIGID/RConn1 -- Ail/RConn1
  AilBrk_C_1_RIGID/LConn2 -- Act/RConn1

== system sm_aileron_actuator_mech_01_ail/Aileron_Att_1/MountR_Att_1/Bracket L ==
  AilBrk_L_1_RIGID : Subsystem  RequirementInfo={} %GIDa_ce070a9c_7322_41b3_bf6d_d36b664da58a
  Bolt LBrk : Subsystem  RequirementInfo={} %GIDa_a0a3e2cc_f66d_443e_95d5_623cb863521b
  Screws LBrk : Subsystem  RequirementInfo={} %GIDa_c6696f74_e323_404b_9422_7ab4f5ca8322
  Ail : PMIOPort  RequirementInfo={} %GIDa_3ce34dae_74e9_427e_9bfc_6eb68b1d18d0  Side=Right
  connections:
  Screws LBrk/LConn1 -- AilBrk_L_1_RIGID/LConn1 -- Bolt LBrk/LConn1
  AilBrk_L_1_RIGID/RConn1 -- Ail/RConn1

== system sm_aileron_actuator_mech_01_ail/Aileron_Att_1/MountR_Att_1/Bracket R ==
  AilBrk_R_1_RIGID : Subsystem  RequirementInfo={} %GIDa_9209cfae_3950_4d35_8f51_34879a5f743d
  Bolt RBrk : Subsystem  RequirementInfo={} %GIDa_95fa86b9_dd90_4c91_8469_433465665610
  Screws RBrk : Subsystem  RequirementInfo={} %GIDa_2a0b16c2_ba5e_4ceb_b728_ef2610ac4ce0
  Ail : PMIOPort  RequirementInfo={} %GIDa_f3b903d8_f1f9_417a_8399_942b19d6788f  Side=Right
  connections:
  Screws RBrk/LConn1 -- AilBrk_R_1_RIGID/LConn1 -- Bolt RBrk/LConn1
  AilBrk_R_1_RIGID/RConn1 -- Ail/RConn1

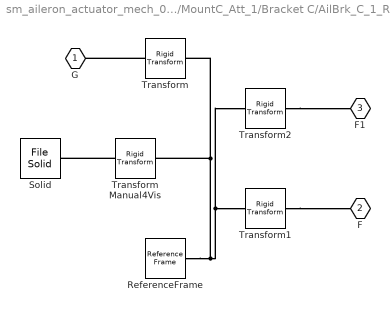
== system sm_aileron_actuator_mech_01_ail/Aileron_Att_1/MountC_Att_1/Bracket C/AilBrk_C_1_RIGID ==
  ReferenceFrame : sm_lib/Frames and Transforms/Reference Frame  RequirementInfo={} %GIDa_ba13444b_e5c2_4f1e_959e_f5dee6569827
  Solid : sm_lib/Body Elements/File Solid  RequirementInfo={} %GIDa_780f2ccf_4e78_4743_851b_df4ee8ad0281  ExtGeomFileName=AilBrk_C.step  UnitType=FromFile  ExtGeomFileUnits=m  StepReaderType=HEX  ExportConvexHullGeometry=off  InertiaType=Custom  Mass=smiData.Solid(15).mass  MassUnits=kg  CenterOfMass=smiData.Solid(15).CoM  CenterOfMassUnits=m  MomentsOfInertia=smiData.Solid(15).MoI  MomentsOfInertiaUnits=kg*m^2  ProductsOfInertia=smiData.Solid(15).PoI  ProductsOfInertiaUnits=kg*m^2  BasedOnType=Density  Density=1000  DensityUnits=kg/m^3  DoExposeReferenceFrame=on  SerializedFrames=<Frames/>  GraphicType=FromGeometry  MarkerShape=Sphere  MarkerSize=10  GraphicVisPropType=SimpleVisualProperties  GraphicDiffuseColor=smiData.Solid(15).color  GraphicSpecularColor=[0.5 0.5 0.5 1.0]  GraphicAmbientColor=[0.15 0.15 0.15 1.0]  GraphicEmissiveColor=[0.0 0.0 0.0 1.0]  GraphicShininess=75  GraphicOpacity=smiData.Solid(15).opacity
  Transform : sm_lib/Frames and Transforms/Rigid Transform  RequirementInfo={} %GIDa_41b926a7_ffda_4999_b67a_7ab78be36583  TranslationMethod=Cartesian  TranslationStandardOffset=0  TranslationStandardOffsetUnits=m  TranslationStandardAxis=+Z  TranslationCartesianOffset=smiData.RigidTransform(98).translation  TranslationCartesianOffsetUnits=m  TranslationROffset=0  TranslationROffsetUnits=m  TranslationZOffset=0  TranslationZOffsetUnits=m  TranslationThetaOffset=0  TranslationThetaOffsetUnits=deg  RotationMethod=ArbitraryAxis  RotationAngleUnits=rad  RotationStandardAxis=+Z  RotationAngle=smiData.RigidTransform(98).angle  RotationArbitraryAxis=smiData.RigidTransform(98).axis  FollAlignAxisA=+X  BaseAlignAxisA=+Y  FollAlignAxisB=+Y  BaseAlignAxisB=+Z  RotationSequenceAxes=FollowerAxes  RotationSequence=XYX  RotationSequenceAngles=[0 0 0]  RotationSequenceAnglesUnits=deg  RotationMatrix=[1 0 0; 0 1 0; 0 0 1]  Quaternion=[1 0 0 0]
  Transform Manual4Vis : sm_lib/Frames and Transforms/Rigid Transform  RequirementInfo={} %GIDa_6ca90dce_e642_4a83_9145_c21aa2d231c8  TranslationMethod=Cartesian  TranslationStandardOffset=0  TranslationStandardOffsetUnits=m  TranslationStandardAxis=+Z  TranslationCartesianOffset=[-1 1 0]*AAC_Param.AilBrk.LRManual4Vis  TranslationCartesianOffsetUnits=m  TranslationROffset=0  TranslationROffsetUnits=m  TranslationZOffset=0  TranslationZOffsetUnits=m  TranslationThetaOffset=0  TranslationThetaOffsetUnits=deg  RotationMethod=None  RotationAngleUnits=deg  RotationStandardAxis=+Z  RotationAngle=0.0  RotationArbitraryAxis=[0 0 1]  FollAlignAxisA=+X  BaseAlignAxisA=+Y  FollAlignAxisB=+Y  BaseAlignAxisB=+Z  RotationSequenceAxes=FollowerAxes  RotationSequence=XYX  RotationSequenceAngles=[0 0 0]  RotationSequenceAnglesUnits=deg  RotationMatrix=[1 0 0; 0 1 0; 0 0 1]  Quaternion=[1 0 0 0]
  Transform1 : sm_lib/Frames and Transforms/Rigid Transform  RequirementInfo={} %GIDa_2d5547e3_fb2d_49af_9696_a6fd5c66b503  TranslationMethod=Cartesian  TranslationStandardOffset=0  TranslationStandardOffsetUnits=m  TranslationStandardAxis=+Z  TranslationCartesianOffset=smiData.RigidTransform(172).translation  TranslationCartesianOffsetUnits=m  TranslationROffset=0  TranslationROffsetUnits=m  TranslationZOffset=0  TranslationZOffsetUnits=m  TranslationThetaOffset=0  TranslationThetaOffsetUnits=deg  RotationMethod=ArbitraryAxis  RotationAngleUnits=rad  RotationStandardAxis=+Z  RotationAngle=smiData.RigidTransform(172).angle  RotationArbitraryAxis=smiData.RigidTransform(172).axis  FollAlignAxisA=+X  BaseAlignAxisA=+Y  FollAlignAxisB=+Y  BaseAlignAxisB=+Z  RotationSequenceAxes=FollowerAxes  RotationSequence=XYX  RotationSequenceAngles=[0 0 0]  RotationSequenceAnglesUnits=deg  RotationMatrix=[1 0 0; 0 1 0; 0 0 1]  Quaternion=[1 0 0 0]
  Transform2 : sm_lib/Frames and Transforms/Rigid Transform  RequirementInfo={} %GIDa_4bed4b42_9ace_4141_b6b4_a6917a116dbe  TranslationMethod=Cartesian  TranslationStandardOffset=0  TranslationStandardOffsetUnits=m  TranslationStandardAxis=+Z  TranslationCartesianOffset=smiData.RigidTransform(200).translation  TranslationCartesianOffsetUnits=m  TranslationROffset=0  TranslationROffsetUnits=m  TranslationZOffset=0  TranslationZOffsetUnits=m  TranslationThetaOffset=0  TranslationThetaOffsetUnits=deg  RotationMethod=ArbitraryAxis  RotationAngleUnits=rad  RotationStandardAxis=+Z  RotationAngle=smiData.RigidTransform(200).angle  RotationArbitraryAxis=smiData.RigidTransform(200).axis  FollAlignAxisA=+X  BaseAlignAxisA=+Y  FollAlignAxisB=+Y  BaseAlignAxisB=+Z  RotationSequenceAxes=FollowerAxes  RotationSequence=XYX  RotationSequenceAngles=[0 0 0]  RotationSequenceAnglesUnits=deg  RotationMatrix=[1 0 0; 0 1 0; 0 0 1]  Quaternion=[1 0 0 0]
  G : PMIOPort  RequirementInfo={} %GIDa_eb9c430f_1306_40c3_9a23_58608d312bf9  Side=Left
  F : PMIOPort  RequirementInfo={} %GIDa_e2137ba4_fd47_40be_9e91_e7b4c710c44a  Port=2  Side=Right
  F1 : PMIOPort  RequirementInfo={} %GIDa_5894cadd_5a1f_47ef_a0c5_bf359856a17a  Port=3  Side=Left
  connections:
  Transform Manual4Vis/RConn1 -- Solid/RConn1
  Transform/LConn1 -- G/RConn1
  Transform1/RConn1 -- F/RConn1
  Transform2/RConn1 -- F1/RConn1
  ReferenceFrame/RConn1 -- Transform1/LConn1 -- Transform2/LConn1 -- Transform Manual4Vis/LConn1 -- Transform/RConn1

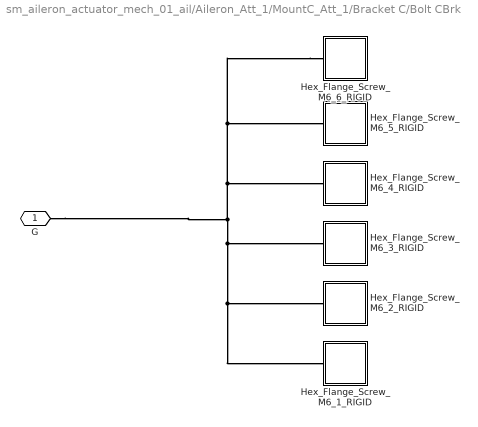
== system sm_aileron_actuator_mech_01_ail/Aileron_Att_1/MountC_Att_1/Bracket C/Bolt CBrk ==
  Hex_Flange_Screw_M6_1_RIGID : Subsystem  RequirementInfo={} %GIDa_3f3bfb32_c03e_434a_a314_69c011d2a633
  Hex_Flange_Screw_M6_2_RIGID : Subsystem  RequirementInfo={} %GIDa_b5eba113_84fd_45a7_89e3_0a7017293c57
  Hex_Flange_Screw_M6_3_RIGID : Subsystem  RequirementInfo={} %GIDa_3ffad671_acba_44d1_ab23_fa626e51bac6
  Hex_Flange_Screw_M6_4_RIGID : Subsystem  RequirementInfo={} %GIDa_4164e3c3_c0c6_4319_bcf7_56c83c61aec5
  Hex_Flange_Screw_M6_5_RIGID : Subsystem  RequirementInfo={} %GIDa_adf00db7_d254_4518_9be1_49c2f454d6b0
  Hex_Flange_Screw_M6_6_RIGID : Subsystem  RequirementInfo={} %GIDa_4e3069d2_0182_4b34_a834_7ec9cff4c96c
  G : PMIOPort  RequirementInfo={} %GIDa_6e5efc2f_0b71_438f_84a3_e90cbdd2b82f  Side=Left
  connections:
  Hex_Flange_Screw_M6_6_RIGID/LConn1 -- Hex_Flange_Screw_M6_5_RIGID/LConn1 -- G/RConn1 -- Hex_Flange_Screw_M6_1_RIGID/LConn1 -- Hex_Flange_Screw_M6_2_RIGID/LConn1 -- Hex_Flange_Screw_M6_3_RIGID/LConn1 -- Hex_Flange_Screw_M6_4_RIGID/LConn1

== system sm_aileron_actuator_mech_01_ail/Aileron_Att_1/MountC_Att_1/Bracket C/Screws CBrk ==
  Hex_Bolt_M10_3_RIGID : Subsystem  RequirementInfo={} %GIDa_36632ab2_0e1a_4787_b5b3_9c3a48aa3cad
  Hex_Flange_Nut_M10_1_RIGID : Subsystem  RequirementInfo={} %GIDa_7b6e3b5f_ba18_4b68_8bf2_3b24c83afeac
  Washer_3_RIGID : Subsystem  RequirementInfo={} %GIDa_68bb6efb_fa03_4a89_ab11_19389535140d
  Washer_4_RIGID : Subsystem  RequirementInfo={} %GIDa_1fab16ed_2885_4e4b_aa7f_78931dd0eeb8
  G : PMIOPort  RequirementInfo={} %GIDa_2d703456_b882_44ab_8b5b_ae85813049d7  Side=Left
  connections:
  Hex_Bolt_M10_3_RIGID/LConn1 -- G/RConn1 -- Washer_4_RIGID/LConn1 -- Washer_3_RIGID/LConn1 -- Hex_Flange_Nut_M10_1_RIGID/LConn1
